simulink model "dsm_v1_no_deci"  (R2025b)
settings: Solver=VariableStepAuto  StartTime=0.0  StopTime=Ts  RelTol=1e-3
undefined symbols (not defined in the file or in its folder): dspblkCoreblockFVToolHelper, gcbh
settings Model: Creator=korvo  LastModifiedBy=korvo

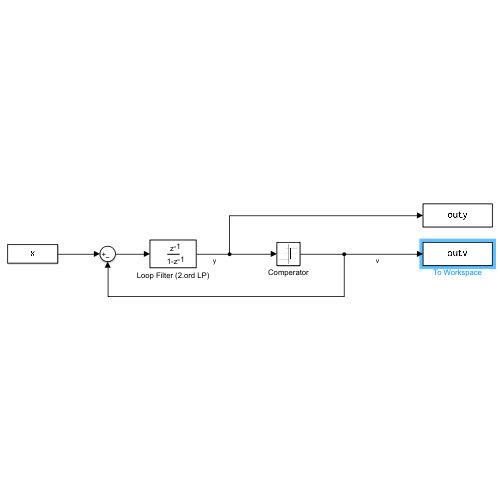
[thumbnail: Simulink's stored preview of the top-level diagram]
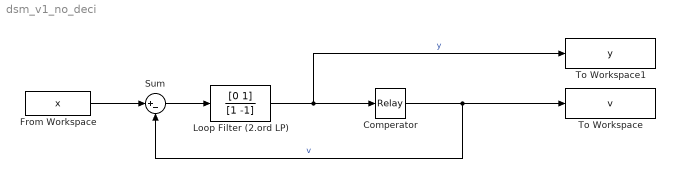
== system dsm_v1_no_deci ==
  Comperator : Relay  OffOutputValue=-1
  From Workspace : FromWorkspace  VariableName=x
  Loop Filter (2.ord LP) : DiscreteFilter  LoadFcn=dspblkCoreblockFVToolHelper(gcbh,'load');  Numerator=[0 1]  Denominator=[1 -1]
      settings: CopyFcn=dspblkCoreblockFVToolHelper(gcbh,'copy');  DeleteFcn=dspblkCoreblockFVToolHelper(gcbh,'close');  ModelCloseFcn=dspblkCoreblockFVToolHelper(gcbh,'close');  PreSaveFcn=dspblkCoreblockFVToolHelper(gcbh,'presave');  PostSaveFcn=dspblkCoreblockFVToolHelper(gcbh,'postsave');  CloseFcn=dspblkCoreblockFVToolHelper(gcbh,'close');
  Sum : Sum  Inputs=|+-
  To Workspace : ToWorkspace  VariableName=v  SampleTime=-1
      settings: Save2DSignal=2-D array (concatenate along first dimension)
  To Workspace1 : ToWorkspace  VariableName=y  SampleTime=-1
      settings: Save2DSignal=2-D array (concatenate along first dimension)
  wires:
  From Workspace/1 -> Sum/1
  Sum/1 -> Loop Filter (2.ord LP)/1
  Loop Filter (2.ord LP)/1 -> To Workspace1/1, Comperator/1  "y"
  Comperator/1 -> Sum/2, To Workspace/1  "v"
